simulink model "LLR_equivalent"  (Simulink 10.0)
settings: Solver=FixedStepDiscrete  StartTime=0.0  StopTime=1  FixedStep=1  RelTol=1e-3  EnableMultiTasking=on
PreLoadFcn:
  | L1 = 1;
  | L2 = 1;
  | R  = 1;
StopFcn:
  | if(0)  % PAS UTILISEE
  | disp('*** Réseau équivalent de type LLR: ***');
  | disp('DONNÉES:');
  | fprintf( '[1] Fondamentale = %2.0f (Hz),  [2] Harmonique(N) = %1.0f,\n',f1,N);
  | fprintf('[3] Impedance fondamentale = %6.3f(Ohms)\n',Mod_Zf1);
  | fprintf('[4] Angle(fondamentale) = %6.2f(deg), Angle(harmonique) = %6.2f(deg)\n',Angle_deg,Angle_N_deg);
  | disp('SOLUTION:')
  | if(d_err)
  | disp('!Remarque: Ne trouve pas de solution.')
  | else
  | fprintf(' R2_llr = %6.4f (Ohms),  L2_llr = %6.3f (mH),  L1_llr =%6.3f (mH)\n\n',R2_llr,L2_llr*1000,L1_llr*1000);
  | disp('NOTE: Pour tracer une réponse en fréquence ouvrir LLR_scan et utilisez la fonction du GUI.');
  | end
  | disp('====')
  | end;
libraries: powerlib x8, simulink x3
settings Model: Creator=Silvano  LastModifiedBy=bhisma
settings DataIOCC: LimitDataPoints=on  SignalLoggingSaveFormat=ModelDataLogs  SaveOutput=off  SaveTime=off
settings OptimizationCC: ExpressionDepthLimit=2147483647  InitFltsAndDblsToZero=on
settings DebuggingCC: AlgebraicLoopMsg=none  SolverPrmCheckMsg=warning  FcnCallInpInsideContextMsg=warning  UnconnectedInputMsg=none  UnconnectedOutputMsg=none  UnconnectedLineMsg=none  StateNameClashWarn=warning
settings GRTTargetCC: GeneratePreprocessorConditionals=Disable all
settings ConfigComp: CovExternalEMLEnable=off
settings SimscapeCC: SimscapeNormalizeSystem=off

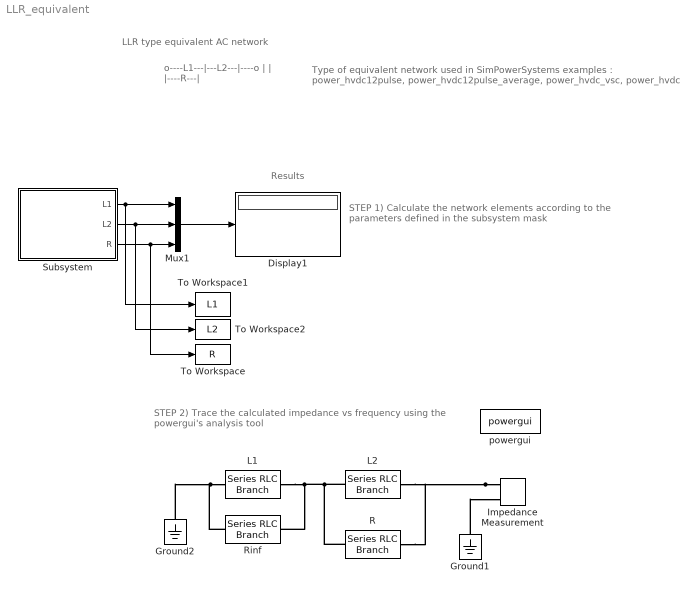
== system LLR_equivalent ==
  note: Type of equivalent network used in SimPowerSystems examples :
      | power_hvdc12pulse, power_hvdc12pulse_average,
      | power_hvdc_vsc, power_hvdc
  note: LLR type equivalent AC network
  note: o----L1---|---L2---|----o
      |                |            |
      |                |----R---|
  note: Results
  note: STEP 2) Trace  the calculated impedance vs frequency
      | using the powergui's analysis tool
  note: STEP 1) Calculate the network elements according
      | to the parameters defined in the subsystem mask
  Display1 : Display
      settings: AttributesFormatString="1) L1 (H)        %<Tag>\\n2) L2 (H)        %<Tag>\\n3) R (ohms)    %<Tag>"  Format=short_e
  Ground1 : powerlib/Elements/Ground  LConnTagsString=a
      settings: SourceProductName=Simscape Electrical
  Ground2 : powerlib/Elements/Ground  LConnTagsString=a
      settings: SourceProductName=Simscape Electrical
  Impedance Measurement : powerlib/Measurements/Impedance Measurement  LConnTagsString=+|-  Factor=1
      settings: SourceProductName=Simscape Electrical  SourceProductBaseCode=PS
  L1 : powerlib/Elements/Series RLC Branch  LConnTagsString=__new0  RConnTagsString=__new0  BranchType=L  Resistance=1  Inductance=L1  SetiL0=off  InitialCurrent=0  Capacitance=1e-6  Setx0=off  InitialVoltage=0  Measurements=None
      settings: SourceProductName=Simscape Electrical
  L2 : powerlib/Elements/Series RLC Branch  LConnTagsString=__new0  RConnTagsString=__new0  BranchType=L  Resistance=1  Inductance=L2  SetiL0=off  InitialCurrent=0  Capacitance=1e-6  Setx0=off  InitialVoltage=0  Measurements=None
      settings: SourceProductName=Simscape Electrical
  Mux1 : Mux  Inputs=3
  R : powerlib/Elements/Series RLC Branch  LConnTagsString=__new0  RConnTagsString=__new0  BranchType=R  Resistance=R  Inductance=1e-3  SetiL0=off  InitialCurrent=0  Capacitance=1e-6  Setx0=off  InitialVoltage=0  Measurements=None
      settings: SourceProductName=Simscape Electrical
  Rinf : powerlib/Elements/Series RLC Branch  LConnTagsString=__new0  RConnTagsString=__new0  BranchType=R  Resistance=1e6  Inductance=1e-3  SetiL0=off  InitialCurrent=0  Capacitance=1e-6  Setx0=off  InitialVoltage=0  Measurements=None
      settings: SourceProductName=Simscape Electrical
  Subsystem : Subsystem  mask(LLR equivalent network calculator){N_f1=60, N_f2=3, Mod_Zf1=500^2/5000, Angle_deg=80}
      mask prompts: N_f1 "Fundemental frequency (Hz):"; N_f2 "Harmonic number (N):"; Mod_Zf1 "Fundamental impedance (Ohms):"; Angle_deg "Phase angle (deg > 0):"
      mask help:
      | Equivalent network : L1 in series with L2//R2
      |
      | The elements L1(H), L2(H), R2(Ohms) are calculated according to the following conditions:
      | 1) The phase angle (deg) is the same for the fundamental frequency (50 or 60 Hz)and the specified harmonic number (N);
      | 2) The fundamental impedance is specified.
      mask init:
      | if (N_f1 == 1)
      |     f1 = 50;
      | else
      |     f1 = 60;
      | end
      | 
      | f2 = (N_f2+1)* f1;
      mask TypeOptions N_f1: 50 | 60
      mask TypeOptions N_f2: 2 | 3 | 4 | 5
      mask Display: disp('LLR network\n calculator')
  To Workspace : ToWorkspace  VariableName=R  SampleTime=-1
      settings: MaxDataPoints=1
  To Workspace1 : ToWorkspace  VariableName=L1  SampleTime=-1
      settings: MaxDataPoints=1
  To Workspace2 : ToWorkspace  VariableName=L2  SampleTime=-1
      settings: MaxDataPoints=1
  powergui : powerlib/powergui  SimulationMode=Discrete  SolverType=Tustin  SampleTime=1  frequency=60  SPID=off  DisableSnubberDevices=off  DisableRonSwitches=off  DisableVfSwitches=off  SwTol=0  Interpol=off  DisplayEquations=off  frequencyindice=60  Pbase=100e6  ErrMax=1e-4  Iterations=50  UnitsV=kV  UnitsW=MW  FunctionMessages=off  echomessages=off  HookPort=off  EnableUseOfTLC=off  x0status=blocks  RestoreLinks=warning  ResistiveCurrentMeasurement=off  Frange=[1:2:500]  Ylog=off  Xlog=off  ShowGrid=on  save=off  variable=ZData  ZoomFFT=on  StartTime=0.0  cycles=1  DisplayStyle=1  fundamental=60  FreqAxis=off  MaxFrequency=1000  frequencyindicesteady=1  RmsSteady=1  display=off  Ts=0  methode=off
      settings: SourceProductName=Simscape Electrical
  wires:
  Mux1/1 -> Display1/1
  Subsystem/1(L1) -> To Workspace1/1, Mux1/1
  Subsystem/2(L2) -> To Workspace2/1, Mux1/2
  Subsystem/3(R) -> To Workspace/1, Mux1/3
  connections:
  L2/LConn1 -- L1/RConn1 -- Rinf/RConn1 -- R/LConn1
  L1/LConn1 -- Rinf/LConn1 -- Ground2/LConn1
  Impedance Measurement/LConn1 -- L2/RConn1 -- R/RConn1
  Ground1/LConn1 -- Impedance Measurement/LConn2

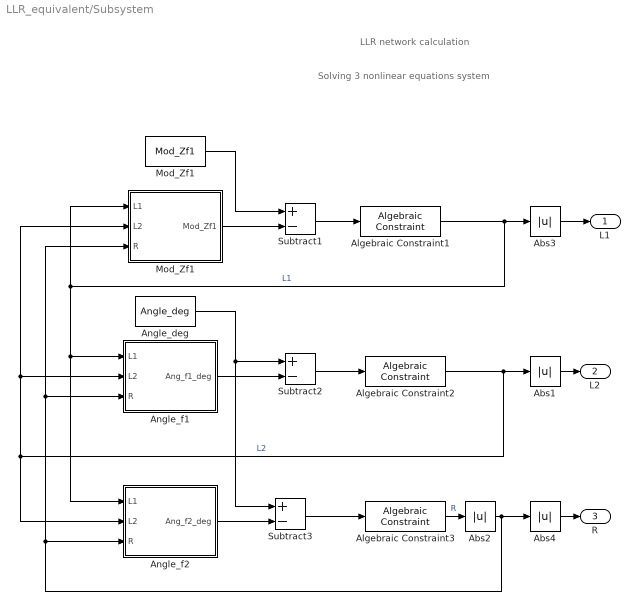
== system LLR_equivalent/Subsystem ==
  note: Solving 3 nonlinear equations system
  note: LLR network calculation
  Abs{1..4} (4 alike) : Abs
  Algebraic Constraint1 : simulink/Math Operations/Algebraic Constraint  z0=Mod_Zf1/(2*pi*f1) *0.4
      settings: SourceProductName=Simulink  SourceProductBaseCode=SL
  Algebraic Constraint2 : simulink/Math Operations/Algebraic Constraint  z0=Mod_Zf1/(2*pi*f1)*0.2
      settings: SourceProductName=Simulink  SourceProductBaseCode=SL
  Algebraic Constraint3 : simulink/Math Operations/Algebraic Constraint  z0=Mod_Zf1*0.3
      settings: SourceProductName=Simulink  SourceProductBaseCode=SL
  Angle_deg : Constant  Value=Angle_deg
  Angle_f1 : Subsystem
  Angle_f2 : Subsystem
  Mod_Zf1 : Constant  Value=Mod_Zf1
  "Mod_Zf1 " : Subsystem
  Subtract1 : Sum  Inputs=+-
  Subtract2 : Sum  Inputs=+-
  Subtract3 : Sum  Inputs=+-
  L1 : Outport
  L2 : Outport  Port=2
  R : Outport  Port=3
  wires:
  Angle_deg/1 -> Subtract3/1, Subtract2/1
  Algebraic Constraint3/1 -> Abs2/1  "R"
  Subtract3/1 -> Algebraic Constraint3/1
  Angle_f2/1(Ang_f2_deg) -> Subtract3/2
  Subtract2/1 -> Algebraic Constraint2/1
  Angle_f1/1(Ang_f1_deg) -> Subtract2/2
  Algebraic Constraint2/1 -> Abs1/1, "Mod_Zf1 "/2(L2), Angle_f1/2(L2), Angle_f2/2(L2)  "L2"
  Algebraic Constraint1/1 -> Abs3/1, "Mod_Zf1 "/1(L1), Angle_f2/1(L1), Angle_f1/1(L1)  "L1"
  Subtract1/1 -> Algebraic Constraint1/1
  Mod_Zf1/1 -> Subtract1/1
  "Mod_Zf1 "/1(Mod_Zf1) -> Subtract1/2
  Abs2/1 -> Abs4/1, "Mod_Zf1 "/3(R), Angle_f1/3(R), Angle_f2/3(R)
  Abs3/1 -> L1/1
  Abs1/1 -> L2/1
  Abs4/1 -> R/1

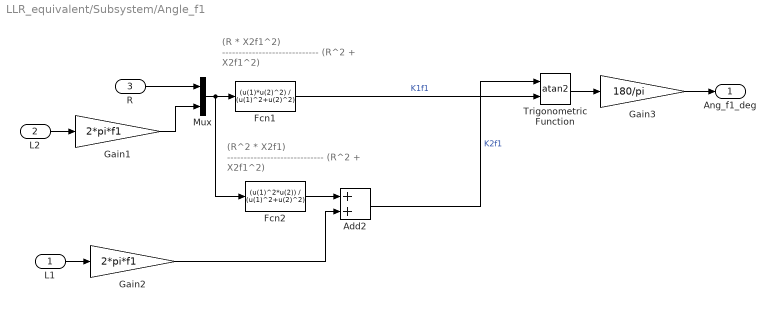
== system LLR_equivalent/Subsystem/Angle_f1 ==
  note: (R * X2f1^2)
      | -----------------------------
      | (R^2 + X2f1^2)
  note: (R^2 * X2f1)
      | -----------------------------
      | (R^2 + X2f1^2)
  L1 : Inport
  L2 : Inport  Port=2
  R : Inport  Port=3
  Add2 : Sum
  Fcn1 : Fcn  Expr=(u(1)*u(2)^2) / (u(1)^2+u(2)^2)
  Fcn2 : Fcn  Expr=(u(1)^2*u(2)) / (u(1)^2+u(2)^2)
  Gain1 : Gain  Gain=2*pi*f1
  Gain2 : Gain  Gain=2*pi*f1
  Gain3 : Gain  Gain=180/pi
  Mux : Mux  Inputs=2
  Trigonometric Function : Trigonometry  Operator=atan2
  Ang_f1_deg : Outport
  wires:
  Fcn1/1 -> Trigonometric Function/2  "K1f1"
  Gain3/1 -> Ang_f1_deg/1
  Trigonometric Function/1 -> Gain3/1
  Mux/1 -> Fcn1/1, Fcn2/1
  Gain1/1 -> Mux/2
  Fcn2/1 -> Add2/1
  Gain2/1 -> Add2/2
  Add2/1 -> Trigonometric Function/1  "K2f1"
  R/1 -> Mux/1
  L2/1 -> Gain1/1
  L1/1 -> Gain2/1

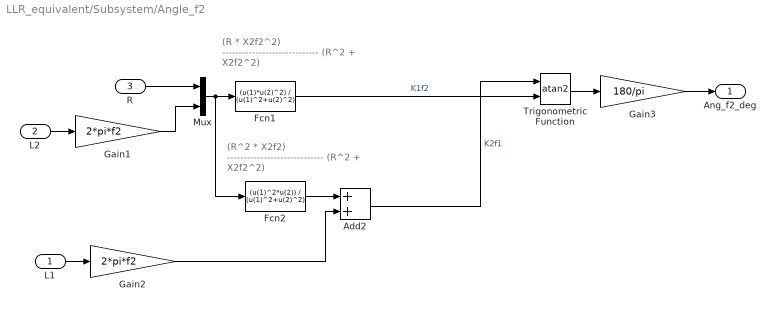
== system LLR_equivalent/Subsystem/Angle_f2 ==
  note: (R^2 * X2f2)
      | -----------------------------
      | (R^2 + X2f2^2)
  note: (R * X2f2^2)
      | -----------------------------
      | (R^2 + X2f2^2)
  L1 : Inport
  L2 : Inport  Port=2
  R : Inport  Port=3
  Add2 : Sum
  Fcn1 : Fcn  Expr=(u(1)*u(2)^2) / (u(1)^2+u(2)^2)
  Fcn2 : Fcn  Expr=(u(1)^2*u(2)) / (u(1)^2+u(2)^2)
  Gain1 : Gain  Gain=2*pi*f2
  Gain2 : Gain  Gain=2*pi*f2
  Gain3 : Gain  Gain=180/pi
  Mux : Mux  Inputs=2
  Trigonometric Function : Trigonometry  Operator=atan2
  Ang_f2_deg : Outport
  wires:
  L1/1 -> Gain2/1
  L2/1 -> Gain1/1
  R/1 -> Mux/1
  Add2/1 -> Trigonometric Function/1  "K2f1"
  Gain2/1 -> Add2/2
  Fcn2/1 -> Add2/1
  Gain1/1 -> Mux/2
  Mux/1 -> Fcn2/1, Fcn1/1
  Trigonometric Function/1 -> Gain3/1
  Gain3/1 -> Ang_f2_deg/1
  Fcn1/1 -> Trigonometric Function/2  "K1f2"

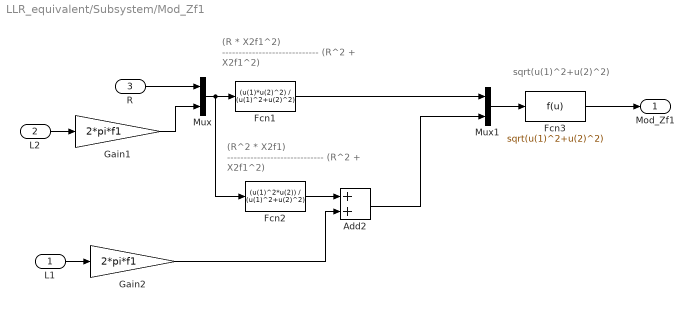
== system LLR_equivalent/Subsystem/Mod_Zf1  ==
  note: sqrt(u(1)^2+u(2)^2)
  note: (R * X2f1^2)
      | -----------------------------
      | (R^2 + X2f1^2)
  note: (R^2 * X2f1)
      | -----------------------------
      | (R^2 + X2f1^2)
  L1 : Inport
  L2 : Inport  Port=2
  R : Inport  Port=3
  Add2 : Sum
  Fcn1 : Fcn  Expr=(u(1)*u(2)^2) / (u(1)^2+u(2)^2)
  Fcn2 : Fcn  Expr=(u(1)^2*u(2)) / (u(1)^2+u(2)^2)
  Fcn3 : Fcn  Expr=sqrt(u(1)^2+u(2)^2)
  Gain1 : Gain  Gain=2*pi*f1
  Gain2 : Gain  Gain=2*pi*f1
  Mux : Mux  Inputs=2
  Mux1 : Mux  Inputs=2
  Mod_Zf1 : Outport
  wires:
  Add2/1 -> Mux1/2
  Fcn1/1 -> Mux1/1
  Mux1/1 -> Fcn3/1
  Mux/1 -> Fcn1/1, Fcn2/1
  Gain1/1 -> Mux/2
  Fcn2/1 -> Add2/1
  Gain2/1 -> Add2/2
  R/1 -> Mux/1
  Fcn3/1 -> Mod_Zf1/1
  L2/1 -> Gain1/1
  L1/1 -> Gain2/1
